simulink model "test_R2017b_latest"  (R2017b)
settings: Solver=VariableStepAuto  StartTime=0.0  StopTime=10  RelTol=1e-3
values from neighbouring files (symbols this model uses):
  A = jacobian([f1,f2, f3, f4], [x1, x2, x3, x4])    [TaylorRemainder.m]    (also in init_ctrl_design.m = eval(A); init_ctrl_design_simple.m = eval(A))
  Ad = eye(4)+A*Ts    [init_ctrl_design.m]    (also in init_ctrl_design_simple.m = eye(2)+A*Ts)
  AK = Ad-Bd*K    [init_ctrl_design.m]    (also in init_ctrl_design_simple.m)
  B = jacobian([f1,f2, f3, f4], [u])    [TaylorRemainder.m]    (also in init_ctrl_design.m = eval(B); init_ctrl_design_simple.m = eval(B); mgcm_acado.m = 1)
  Bd = Ts*B    [init_ctrl_design.m]    (also in init_ctrl_design_simple.m)
  beta = 1    [TaylorRemainder.m]    (also in init_ctrl_design.m; init_ctrl_design_simple.m; solveMGCM.m)
  C = eye(4)    [init_ctrl_design.m]    (also in init_ctrl_design_simple.m = eye(2))
  Cd = eye(4)    [init_ctrl_design.m]    (also in init_ctrl_design_simple.m = eye(2))
  D = zeros(4,1)    [init_ctrl_design.m]    (also in init_ctrl_design_simple.m = zeros(2,1))
  Dd = D    [init_ctrl_design.m]    (also in init_ctrl_design_simple.m)
  init_cond = [x1-0.35, x2-0.4, x3, 0]    [TaylorRemainder.m]    (also in init_ctrl_design.m; init_ctrl_design_simple.m = [x1-0.35, x2-0.4])
  ksi = 1/sqrt(2)    [init_ctrl_design.m]    (also in solveMGCM.m)
  Ts = 0.01    [APRBSgeneration.m]    (also in draw.m; drawCP.m = 0.1; genTrainingData.m = 0.1; init_ctrl_design.m)
  wn = sqrt(1000)    [TaylorRemainder.m]    (also in init_ctrl_design.m; solveMGCM.m)
  x2_c = 0    [TaylorRemainder.m]    (also in init_ctrl_design.m; init_ctrl_design_simple.m; solveMGCM.m)
undefined symbols (not defined in the file or in its folder): DiscIntNeverNeededParam, K
settings Model: Creator=pbevanda  LastModifiedBy=petar
settings SFSimCC: SimUseLocalCustomCode=on
settings RTWCC: RTWUseLocalCustomCode=on

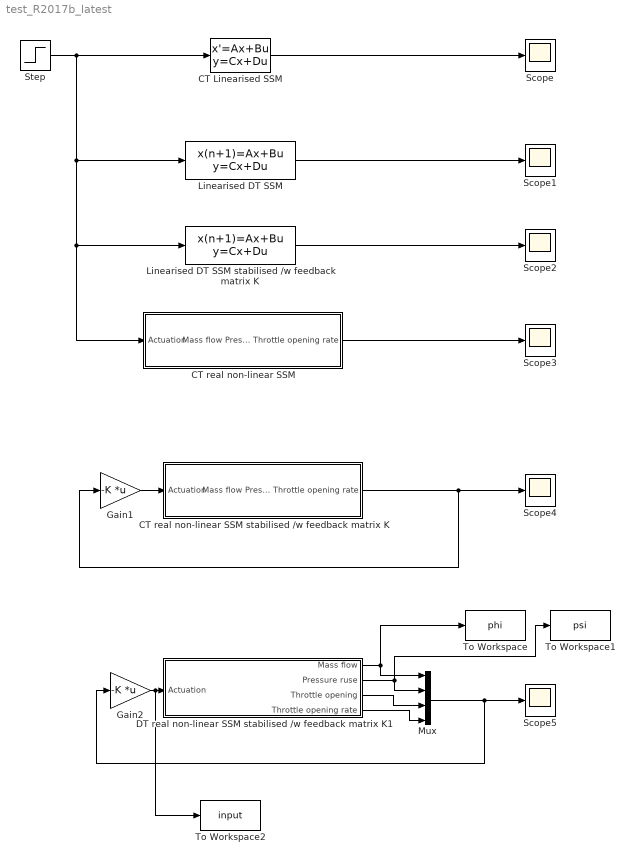
== system test_R2017b_latest ==
  CT Linearised SSM : StateSpace  A=A  B=B  C=C  D=D  InitialCondition=init_cond
  "CT real non-linear SSM " : Subsystem
  CT real non-linear SSM stabilised /w feedback matrix K : Subsystem
  DT real non-linear SSM stabilised /w feedback matrix K1 : Subsystem
  Gain1 : Gain  Gain=-K  Multiplication=Matrix(K*u)
  Gain2 : Gain  Gain=-K  Multiplication=Matrix(K*u)
  "Linearised DT SSM " : DiscreteStateSpace  A=Ad  B=Bd  C=Cd  D=Dd  InitialCondition=init_cond  SampleTime=Ts
  Linearised DT SSM stabilised /w feedback matrix K : DiscreteStateSpace  A=AK  B=zeros(4,1)  C=Cd  D=Dd  InitialCondition=init_cond  SampleTime=Ts
  Mux : Mux
  Scope{,1..5} (6 alike) : Scope
  Step : Step  Time=0  After=0  SampleTime=0
  To Workspace : ToWorkspace  VariableName=phi  SaveFormat=Timeseries  SampleTime=-1
  To Workspace1 : ToWorkspace  VariableName=psi  SaveFormat=Timeseries  SampleTime=-1
  To Workspace2 : ToWorkspace  VariableName=input  SaveFormat=Timeseries  SampleTime=-1
  wires:
  CT Linearised SSM/1 -> Scope/1
  "Linearised DT SSM "/1 -> Scope1/1
  Linearised DT SSM stabilised /w feedback matrix K/1 -> Scope2/1
  "CT real non-linear SSM "/1("Mass flow Pressure ruse Throttle opening Throttle opening rate ") -> Scope3/1
  Step/1 -> "CT real non-linear SSM "/1("Actuation "), Linearised DT SSM stabilised /w feedback matrix K/1, "Linearised DT SSM "/1, CT Linearised SSM/1
  Gain1/1 -> CT real non-linear SSM stabilised /w feedback matrix K/1("Actuation ")
  CT real non-linear SSM stabilised /w feedback matrix K/1("Mass flow Pressure ruse Throttle opening Throttle opening rate ") -> Gain1/1, Scope4/1
  DT real non-linear SSM stabilised /w feedback matrix K1/1("Mass flow ") -> Mux/1, To Workspace/1
  DT real non-linear SSM stabilised /w feedback matrix K1/2("Pressure ruse ") -> Mux/2, To Workspace1/1
  DT real non-linear SSM stabilised /w feedback matrix K1/3("Throttle opening ") -> Mux/3
  DT real non-linear SSM stabilised /w feedback matrix K1/4("Throttle opening rate ") -> Mux/4
  Mux/1 -> Gain2/1, Scope5/1
  Gain2/1 -> To Workspace2/1, DT real non-linear SSM stabilised /w feedback matrix K1/1("Actuation ")

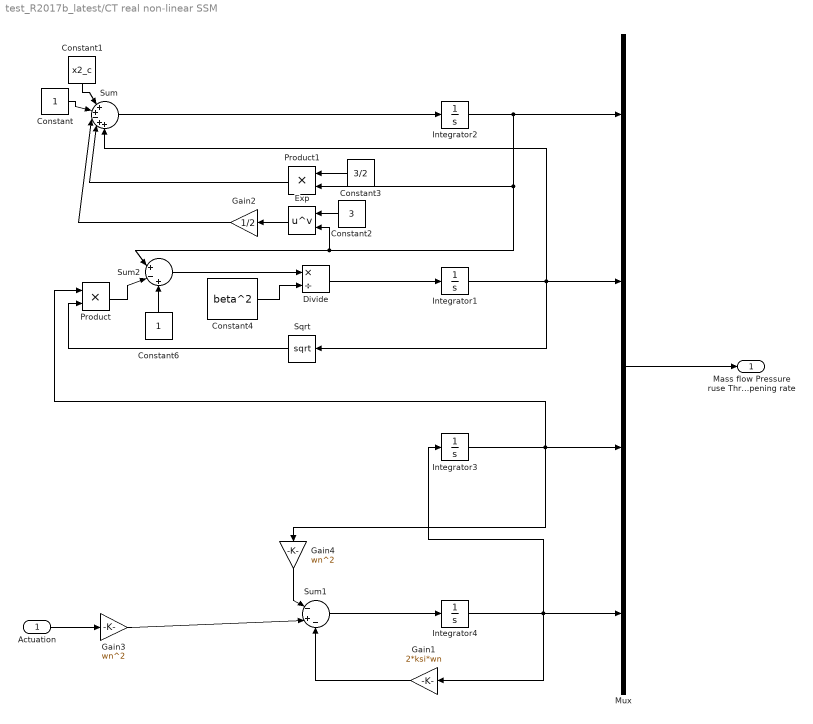
== system test_R2017b_latest/CT real non-linear SSM  ==
  "Actuation " : Inport
  Constant : Constant
  Constant1 : Constant  Value=x2_c
  Constant2 : Constant  Value=3
  Constant3 : Constant  Value=3/2
  Constant4 : Constant  Value=beta^2
  Constant6 : Constant
  Divide : Product  Inputs=*/
  Exp : Math  Operator=pow  SaturateOnIntegerOverflow=on
  Gain1 : Gain  Gain=2*ksi*wn
  Gain2 : Gain  Gain=1/2
  Gain3 : Gain  Gain=wn^2
  Gain4 : Gain  Gain=wn^2
  Integrator1 : Integrator  InitialCondition=init_cond(2)
  Integrator2 : Integrator  InitialCondition=init_cond(1)
  Integrator3 : Integrator  InitialCondition=init_cond(3)
  Integrator4 : Integrator  InitialCondition=init_cond(4)
  Mux : Mux
  Product : Product
  Product1 : Product
  Sqrt : Sqrt  SaturateOnIntegerOverflow=on
  Sum : Sum  Inputs=|++-++
  Sum1 : Sum  Inputs=|-+-
  Sum2 : Sum  Inputs=|+-+
  "Mass flow Pressure ruse Throttle opening Throttle opening rate " : Outport
  wires:
  Mux/1 -> "Mass flow Pressure ruse Throttle opening Throttle opening rate "/1
  Constant/1 -> Sum/2
  Constant1/1 -> Sum/1
  Constant2/1 -> Exp/1
  Constant4/1 -> Divide/2
  Sum2/1 -> Divide/1
  Integrator1/1 -> Sum/5, Mux/2, Sqrt/1
  Integrator2/1 -> Exp/2, Sum2/1, Product1/2, Mux/1
  Constant6/1 -> Sum2/3
  Sqrt/1 -> Product/2
  Product/1 -> Sum2/2
  Divide/1 -> Integrator1/1
  Exp/1 -> Gain2/1
  Gain2/1 -> Sum/3
  Sum/1 -> Integrator2/1
  Constant3/1 -> Product1/1
  Product1/1 -> Sum/4
  Integrator3/1 -> Gain4/1, Product/1, Mux/3
  Integrator4/1 -> Gain1/1, Integrator3/1, Mux/4
  "Actuation "/1 -> Gain3/1
  Sum1/1 -> Integrator4/1
  Gain1/1 -> Sum1/3
  Gain4/1 -> Sum1/1
  Gain3/1 -> Sum1/2

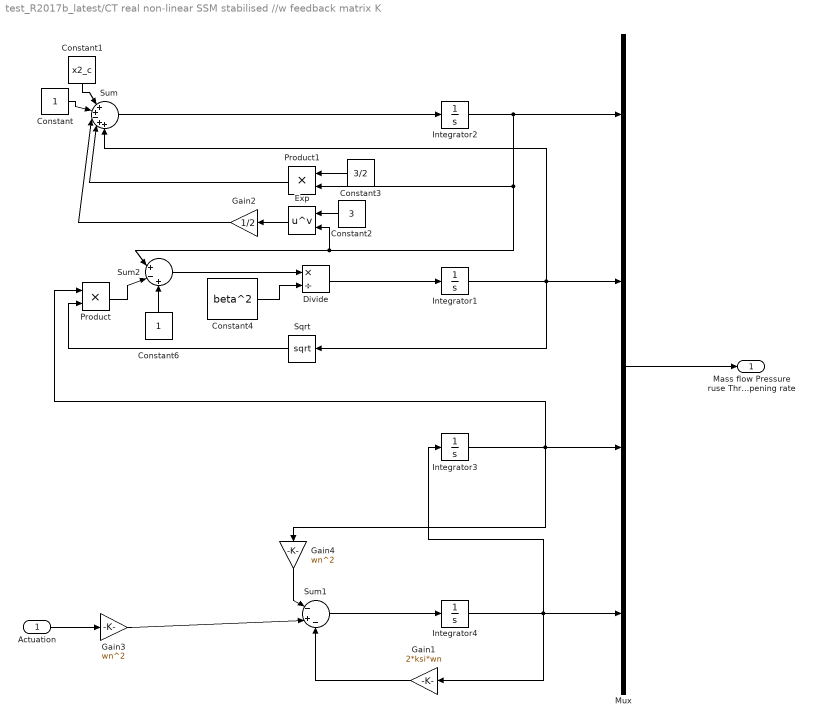
== system test_R2017b_latest/CT real non-linear SSM stabilised //w feedback matrix K ==
  "Actuation " : Inport
  Constant : Constant
  Constant1 : Constant  Value=x2_c
  Constant2 : Constant  Value=3
  Constant3 : Constant  Value=3/2
  Constant4 : Constant  Value=beta^2
  Constant6 : Constant
  Divide : Product  Inputs=*/
  Exp : Math  Operator=pow  SaturateOnIntegerOverflow=on
  Gain1 : Gain  Gain=2*ksi*wn
  Gain2 : Gain  Gain=1/2
  Gain3 : Gain  Gain=wn^2
  Gain4 : Gain  Gain=wn^2
  Integrator1 : Integrator  InitialCondition=init_cond(2)
  Integrator2 : Integrator  InitialCondition=init_cond(1)
  Integrator3 : Integrator  InitialCondition=init_cond(3)
  Integrator4 : Integrator  InitialCondition=init_cond(4)
  Mux : Mux
  Product : Product
  Product1 : Product
  Sqrt : Sqrt  SaturateOnIntegerOverflow=on
  Sum : Sum  Inputs=|++-++
  Sum1 : Sum  Inputs=|-+-
  Sum2 : Sum  Inputs=|+-+
  "Mass flow Pressure ruse Throttle opening Throttle opening rate " : Outport
  wires:
  Mux/1 -> "Mass flow Pressure ruse Throttle opening Throttle opening rate "/1
  Constant/1 -> Sum/2
  Constant1/1 -> Sum/1
  Constant2/1 -> Exp/1
  Constant4/1 -> Divide/2
  Sum2/1 -> Divide/1
  Integrator1/1 -> Sum/5, Mux/2, Sqrt/1
  Integrator2/1 -> Exp/2, Sum2/1, Product1/2, Mux/1
  Constant6/1 -> Sum2/3
  Sqrt/1 -> Product/2
  Product/1 -> Sum2/2
  Divide/1 -> Integrator1/1
  Exp/1 -> Gain2/1
  Gain2/1 -> Sum/3
  Sum/1 -> Integrator2/1
  Constant3/1 -> Product1/1
  Product1/1 -> Sum/4
  Integrator3/1 -> Gain4/1, Product/1, Mux/3
  Integrator4/1 -> Gain1/1, Integrator3/1, Mux/4
  "Actuation "/1 -> Gain3/1
  Sum1/1 -> Integrator4/1
  Gain1/1 -> Sum1/3
  Gain4/1 -> Sum1/1
  Gain3/1 -> Sum1/2

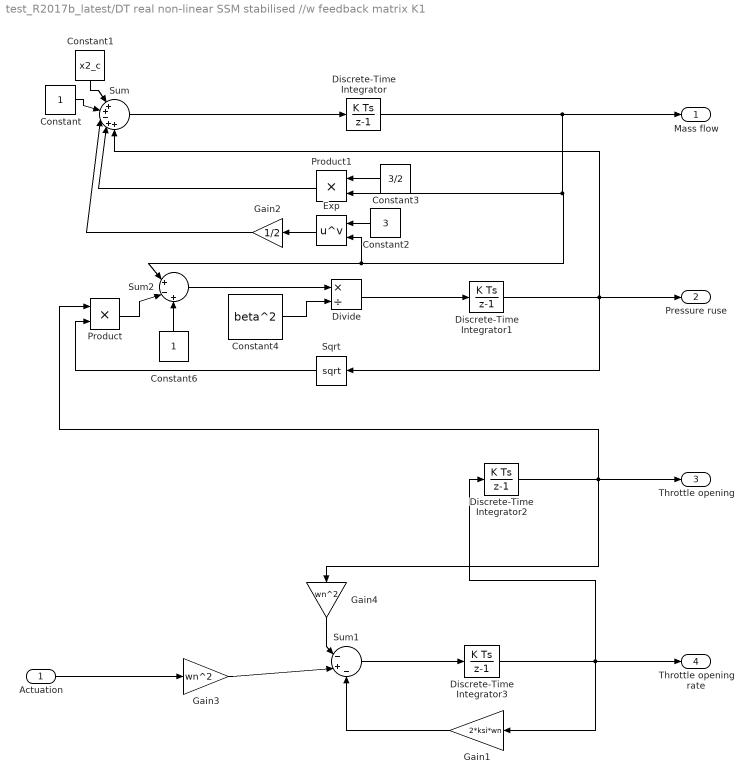
== system test_R2017b_latest/DT real non-linear SSM stabilised //w feedback matrix K1 ==
  "Actuation " : Inport
  Constant : Constant
  Constant1 : Constant  Value=x2_c
  Constant2 : Constant  Value=3
  Constant3 : Constant  Value=3/2
  Constant4 : Constant  Value=beta^2
  Constant6 : Constant
  Discrete-Time Integrator : DiscreteIntegrator  InitialCondition=init_cond(1)  InitialConditionSetting=State (most efficient)  SampleTime=-1  ICPrevOutput=DiscIntNeverNeededParam  ICPrevScaledInput=DiscIntNeverNeededParam
  Discrete-Time Integrator1 : DiscreteIntegrator  InitialCondition=init_cond(2)  InitialConditionSetting=State (most efficient)  SampleTime=-1  ICPrevOutput=DiscIntNeverNeededParam  ICPrevScaledInput=DiscIntNeverNeededParam
  Discrete-Time Integrator2 : DiscreteIntegrator  InitialCondition=init_cond(3)  InitialConditionSetting=State (most efficient)  SampleTime=-1  ICPrevOutput=DiscIntNeverNeededParam  ICPrevScaledInput=DiscIntNeverNeededParam
  Discrete-Time Integrator3 : DiscreteIntegrator  InitialCondition=init_cond(4)  InitialConditionSetting=State (most efficient)  SampleTime=-1  ICPrevOutput=DiscIntNeverNeededParam  ICPrevScaledInput=DiscIntNeverNeededParam
  Divide : Product  Inputs=*/
  Exp : Math  Operator=pow  SaturateOnIntegerOverflow=on
  Gain1 : Gain  Gain=2*ksi*wn
  Gain2 : Gain  Gain=1/2
  Gain3 : Gain  Gain=wn^2
  Gain4 : Gain  Gain=wn^2
  Product : Product
  Product1 : Product
  Sqrt : Sqrt  SaturateOnIntegerOverflow=on
  Sum : Sum  Inputs=|++-++
  Sum1 : Sum  Inputs=|-+-
  Sum2 : Sum  Inputs=|+-+
  "Mass flow " : Outport
  "Pressure ruse " : Outport  Port=2
  "Throttle opening " : Outport  Port=3
  "Throttle opening rate " : Outport  Port=4
  wires:
  Constant/1 -> Sum/2
  Constant1/1 -> Sum/1
  Constant2/1 -> Exp/1
  Constant4/1 -> Divide/2
  Sum2/1 -> Divide/1
  Constant6/1 -> Sum2/3
  Sqrt/1 -> Product/2
  Product/1 -> Sum2/2
  Divide/1 -> Discrete-Time Integrator1/1
  Exp/1 -> Gain2/1
  Gain2/1 -> Sum/3
  Constant3/1 -> Product1/1
  Product1/1 -> Sum/4
  Sum1/1 -> Discrete-Time Integrator3/1
  Gain1/1 -> Sum1/3
  Gain4/1 -> Sum1/1
  Sum/1 -> Discrete-Time Integrator/1
  Gain3/1 -> Sum1/2
  "Actuation "/1 -> Gain3/1
  Discrete-Time Integrator2/1 -> "Throttle opening "/1, Gain4/1, Product/1
  Discrete-Time Integrator3/1 -> "Throttle opening rate "/1, Discrete-Time Integrator2/1, Gain1/1
  Discrete-Time Integrator/1 -> "Mass flow "/1, Product1/2, Exp/2, Sum2/1
  Discrete-Time Integrator1/1 -> "Pressure ruse "/1, Sum/5, Sqrt/1
